simulink model "delay_test"  (R2019a)
settings: Solver=VariableStepAuto  StartTime=0.0  StopTime=512  RelTol=1e-3
libraries: xbsIndex_r4 x3559
(part 3 of 23)

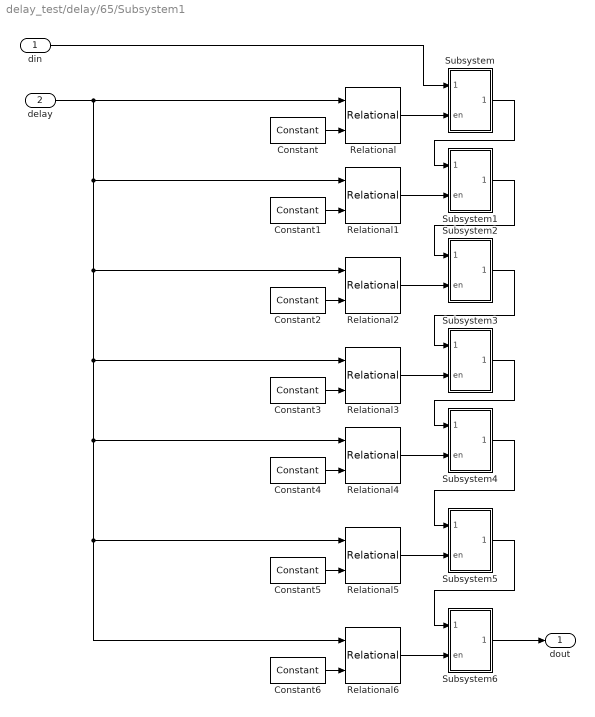
== system delay_test/delay/65/Subsystem1 ==
  din : Inport
  delay : Inport  Port=2
  Constant : xbsIndex_r4/Constant  const=0  gui_display_data_type=Fixed-point  arith_type=Unsigned  n_bits=3  bin_pt=0  preci_type=Single  exp_width=8  frac_width=24  explicit_period=on  period=1  equ=P=C  opselect=C  inp2=PCIN>>17  opr=+  inp1=P  carry=CIN  dbl_ovrd=off  block_type=constant
  Constant1 : xbsIndex_r4/Constant  const=1  gui_display_data_type=Fixed-point  arith_type=Unsigned  n_bits=3  bin_pt=0  preci_type=Single  exp_width=8  frac_width=24  explicit_period=on  period=1  equ=P=C  opselect=C  inp2=PCIN>>17  opr=+  inp1=P  carry=CIN  dbl_ovrd=off  block_type=constant
  Constant2 : xbsIndex_r4/Constant  const=2  gui_display_data_type=Fixed-point  arith_type=Unsigned  n_bits=3  bin_pt=0  preci_type=Single  exp_width=8  frac_width=24  explicit_period=on  period=1  equ=P=C  opselect=C  inp2=PCIN>>17  opr=+  inp1=P  carry=CIN  dbl_ovrd=off  block_type=constant
  Constant3 : xbsIndex_r4/Constant  const=3  gui_display_data_type=Fixed-point  arith_type=Unsigned  n_bits=3  bin_pt=0  preci_type=Single  exp_width=8  frac_width=24  explicit_period=on  period=1  equ=P=C  opselect=C  inp2=PCIN>>17  opr=+  inp1=P  carry=CIN  dbl_ovrd=off  block_type=constant
  Constant4 : xbsIndex_r4/Constant  const=4  gui_display_data_type=Fixed-point  arith_type=Unsigned  n_bits=3  bin_pt=0  preci_type=Single  exp_width=8  frac_width=24  explicit_period=on  period=1  equ=P=C  opselect=C  inp2=PCIN>>17  opr=+  inp1=P  carry=CIN  dbl_ovrd=off  block_type=constant
  Constant5 : xbsIndex_r4/Constant  const=5  gui_display_data_type=Fixed-point  arith_type=Unsigned  n_bits=3  bin_pt=0  preci_type=Single  exp_width=8  frac_width=24  explicit_period=on  period=1  equ=P=C  opselect=C  inp2=PCIN>>17  opr=+  inp1=P  carry=CIN  dbl_ovrd=off  block_type=constant
  Constant6 : xbsIndex_r4/Constant  const=6  gui_display_data_type=Fixed-point  arith_type=Unsigned  n_bits=3  bin_pt=0  preci_type=Single  exp_width=8  frac_width=24  explicit_period=on  period=1  equ=P=C  opselect=C  inp2=PCIN>>17  opr=+  inp1=P  carry=CIN  dbl_ovrd=off  block_type=constant
  Relational{,1..6} (7 alike) : xbsIndex_r4/Relational  mode=a>b  op_type=Bool  en=off  latency=1  dbl_ovrd=off  block_type=relational
  Subsystem : Subsystem
  Subsystem1 : Subsystem
  Subsystem2 : Subsystem
  Subsystem3 : Subsystem
  Subsystem4 : Subsystem
  Subsystem5 : Subsystem
  Subsystem6 : Subsystem
  dout : Outport
  wires:
  Constant3/1 -> Relational3/2
  Constant6/1 -> Relational6/2
  Constant1/1 -> Relational1/2
  Relational/1 -> Subsystem/2(en)
  Constant5/1 -> Relational5/2
  Relational1/1 -> Subsystem1/2(en)
  delay/1 -> Relational6/1, Relational5/1, Relational4/1, Relational3/1, Relational2/1, Relational1/1, Relational/1
  Constant4/1 -> Relational4/2
  Relational4/1 -> Subsystem4/2(en)
  Relational2/1 -> Subsystem2/2(en)
  Relational6/1 -> Subsystem6/2(en)
  Constant/1 -> Relational/2
  Relational5/1 -> Subsystem5/2(en)
  Relational3/1 -> Subsystem3/2(en)
  Constant2/1 -> Relational2/2
  Subsystem6/1(dout) -> dout/1
  Subsystem4/1(dout) -> Subsystem5/1(din)
  Subsystem5/1(dout) -> Subsystem6/1(din)
  Subsystem3/1(dout) -> Subsystem4/1(din)
  Subsystem2/1(dout) -> Subsystem3/1(din)
  Subsystem1/1(dout) -> Subsystem2/1(din)
  Subsystem/1(dout) -> Subsystem1/1(din)
  din/1 -> Subsystem/1(din)

== system delay_test/delay/65/delay ==
  sim_1 : Inport
  io_delay : xbsIndex_r4/Delay  rst=off  infoeditControl=Selection of Reset will increase slice count due to use of real FFs and instead of SRLs  en=off  latency=0  reg_retiming=on  dbl_ovrd=off  block_type=delay
  reint1 : xbsIndex_r4/Reinterpret  force_arith_type=on  arith_type=Unsigned  force_bin_pt=on  bin_pt=0  block_type=reinterpret
  slice_reg : xbsIndex_r4/Slice  nbits=13  boolean_output=off  mode=Lower Bit Location + Width  bit1=0  base1=MSB of Input  bit0=0  base0=LSB of Input  dbl_ovrd=off  block_type=slice
  snap2_f_200msps_64i_4096c_delay_0_delay_user_data_out : xbsIndex_r4/Gateway In  gui_display_data_type=Fixed-point  arith_type=Unsigned  n_bits=32  bin_pt=0  preci_type=Single  exp_width=8  frac_width=24  rows=1  columns=1  quantization="Round  (unbiased: +/- Inf)"  overflow=Saturate  period=1  UseAsADC=off  ADCChannel='1'  interface=None  automatic_assignment=on  address_offset=hex2dec('00')  intf_name=''  intf_description=''  default_value=0  timing_constraint=None  locs_specified=off  LOCs={}  io_standard={}  inherit_from_input=off  hdl_port=on  dbl_ovrd=off  block_type=gatewayin
  in_reg : Outport
  wires:
  reint1/1 -> in_reg/1
  slice_reg/1 -> reint1/1
  io_delay/1 -> slice_reg/1
  ? -> snap2_f_200msps_64i_4096c_delay_0_delay_user_data_out/1
  ? -> ?
  ? -> ?
  sim_1/1 -> ?
  snap2_f_200msps_64i_4096c_delay_0_delay_user_data_out/1 -> io_delay/1

== system delay_test/delay/65/delay_bram_prog_dp ==
  din : Inport
  delay : Inport  Port=2
  AddSub : xbsIndex_r4/AddSub  mode=Subtraction  use_carryin=off  use_carryout=off  en=off  latency=1  precision=User Defined  arith_type=Unsigned  n_bits=ram_bits  bin_pt=0  quantization=Truncate  overflow=Wrap  use_behavioral_HDL=on  hw_selection=Fabric  pipelined=off  use_rpm=on  dbl_ovrd=off  block_type=addsub
  Constant2 : xbsIndex_r4/Constant  const=1.0  gui_display_data_type=Fixed-point  arith_type=Boolean  n_bits=1  bin_pt=0  preci_type=Single  exp_width=8  frac_width=24  explicit_period=on  period=1  equ=P=C  opselect=C  inp2=PCIN>>17  opr=+  inp1=P  carry=CIN  dbl_ovrd=off  block_type=constant
  Constant4 : xbsIndex_r4/Constant  const=0  gui_display_data_type=Fixed-point  arith_type=Boolean  n_bits=1  bin_pt=0  preci_type=Single  exp_width=8  frac_width=24  explicit_period=on  period=1  equ=P=C  opselect=C  inp2=PCIN>>17  opr=+  inp1=P  carry=CIN  dbl_ovrd=off  block_type=constant
  Dual Port RAM : xbsIndex_r4/Dual Port RAM  depth=2^ram_bits  initVector=0  distributed_mem=Block RAM  init_a=0  init_b=0  rst_a=off  rst_b=off  en_a=off  en_b=off  latency=bram_latency  write_mode_A=Read After Write  write_mode_B=Read Before Write  optimize=Area  dbl_ovrd=off  block_type=dpram
  Terminator : Terminator
  wr_addr : xbsIndex_r4/Counter  cnt_type=Free Running  cnt_to=Inf  operation=Up  start_count=0  cnt_by_val=1  arith_type=Unsigned  n_bits=ram_bits  bin_pt=0  load_pin=off  rst=off  en=off  explicit_period=on  period=1  use_behavioral_HDL=on  implementation=Fabric  use_rpm=on  dbl_ovrd=off  block_type=counter
  dout : Outport
  wires:
  Dual Port RAM/2 -> dout/1
  Dual Port RAM/1 -> Terminator/1
  Constant4/1 -> Dual Port RAM/6
  Constant2/1 -> Dual Port RAM/3
  AddSub/1 -> Dual Port RAM/4
  din/1 -> Dual Port RAM/5, Dual Port RAM/2
  wr_addr/1 -> Dual Port RAM/1, AddSub/1
  delay/1 -> AddSub/2

== system delay_test/delay/Subsystem/0 ==
  din : Inport
  delay : Inport  Port=2
  Slice : xbsIndex_r4/Slice  nbits=10  boolean_output=off  mode=Lower Bit Location + Width  bit1=0  base1=MSB of Input  bit0=0  base0=LSB of Input  dbl_ovrd=off  block_type=slice
  Slice1 : xbsIndex_r4/Slice  nbits=3  boolean_output=off  mode=Lower Bit Location + Width  bit1=0  base1=MSB of Input  bit0=10  base0=LSB of Input  dbl_ovrd=off  block_type=slice
  Subsystem1 : Subsystem
  delay_bram_prog_dp : Subsystem  AncestorBlock=casper_library_delays/delay_bram_prog_dp  mask(delay_bram_prog_dp){ram_bits=max_delay_bits-3, bram_latency=2, async=off}
      mask prompts: ram_bits "Max delay (2^?)"; bram_latency "BRAM latency"; async "asynchronous operation"
      mask init:
      | delay_bram_prog_dp_init(gcb, ...
      |     'ram_bits', ram_bits, ...
      |     'bram_latency', bram_latency, ...
      |     'async', async);
  dout : Outport
  wires:
  Subsystem1/1(dout) -> dout/1
  delay_bram_prog_dp/1(dout) -> Subsystem1/1(din)
  Slice1/1 -> Subsystem1/2(delay)
  Slice/1 -> delay_bram_prog_dp/2(delay)
  delay/1 -> Slice/1, Slice1/1
  din/1 -> delay_bram_prog_dp/1(din)

== system delay_test/delay/Subsystem/1 ==
  din : Inport
  delay : Inport  Port=2
  Slice : xbsIndex_r4/Slice  nbits=10  boolean_output=off  mode=Lower Bit Location + Width  bit1=0  base1=MSB of Input  bit0=0  base0=LSB of Input  dbl_ovrd=off  block_type=slice
  Slice1 : xbsIndex_r4/Slice  nbits=3  boolean_output=off  mode=Lower Bit Location + Width  bit1=0  base1=MSB of Input  bit0=10  base0=LSB of Input  dbl_ovrd=off  block_type=slice
  Subsystem1 : Subsystem
  delay_bram_prog_dp : Subsystem  AncestorBlock=casper_library_delays/delay_bram_prog_dp  mask(delay_bram_prog_dp){ram_bits=max_delay_bits-3, bram_latency=2, async=off}
      mask prompts: ram_bits "Max delay (2^?)"; bram_latency "BRAM latency"; async "asynchronous operation"
      mask init:
      | delay_bram_prog_dp_init(gcb, ...
      |     'ram_bits', ram_bits, ...
      |     'bram_latency', bram_latency, ...
      |     'async', async);
  dout : Outport
  wires:
  din/1 -> delay_bram_prog_dp/1(din)
  delay/1 -> Slice1/1, Slice/1
  Slice/1 -> delay_bram_prog_dp/2(delay)
  Slice1/1 -> Subsystem1/2(delay)
  delay_bram_prog_dp/1(dout) -> Subsystem1/1(din)
  Subsystem1/1(dout) -> dout/1

== system delay_test/delay/Subsystem/10 ==
  din : Inport
  delay : Inport  Port=2
  Slice : xbsIndex_r4/Slice  nbits=10  boolean_output=off  mode=Lower Bit Location + Width  bit1=0  base1=MSB of Input  bit0=0  base0=LSB of Input  dbl_ovrd=off  block_type=slice
  Slice1 : xbsIndex_r4/Slice  nbits=3  boolean_output=off  mode=Lower Bit Location + Width  bit1=0  base1=MSB of Input  bit0=10  base0=LSB of Input  dbl_ovrd=off  block_type=slice
  Subsystem1 : Subsystem
  delay_bram_prog_dp : Subsystem  AncestorBlock=casper_library_delays/delay_bram_prog_dp  mask(delay_bram_prog_dp){ram_bits=max_delay_bits-3, bram_latency=2, async=off}
      mask prompts: ram_bits "Max delay (2^?)"; bram_latency "BRAM latency"; async "asynchronous operation"
      mask init:
      | delay_bram_prog_dp_init(gcb, ...
      |     'ram_bits', ram_bits, ...
      |     'bram_latency', bram_latency, ...
      |     'async', async);
  dout : Outport
  wires:
  Subsystem1/1(dout) -> dout/1
  delay_bram_prog_dp/1(dout) -> Subsystem1/1(din)
  Slice1/1 -> Subsystem1/2(delay)
  Slice/1 -> delay_bram_prog_dp/2(delay)
  delay/1 -> Slice/1, Slice1/1
  din/1 -> delay_bram_prog_dp/1(din)

== system delay_test/delay/Subsystem/11 ==
  din : Inport
  delay : Inport  Port=2
  Slice : xbsIndex_r4/Slice  nbits=10  boolean_output=off  mode=Lower Bit Location + Width  bit1=0  base1=MSB of Input  bit0=0  base0=LSB of Input  dbl_ovrd=off  block_type=slice
  Slice1 : xbsIndex_r4/Slice  nbits=3  boolean_output=off  mode=Lower Bit Location + Width  bit1=0  base1=MSB of Input  bit0=10  base0=LSB of Input  dbl_ovrd=off  block_type=slice
  Subsystem1 : Subsystem
  delay_bram_prog_dp : Subsystem  AncestorBlock=casper_library_delays/delay_bram_prog_dp  mask(delay_bram_prog_dp){ram_bits=max_delay_bits-3, bram_latency=2, async=off}
      mask prompts: ram_bits "Max delay (2^?)"; bram_latency "BRAM latency"; async "asynchronous operation"
      mask init:
      | delay_bram_prog_dp_init(gcb, ...
      |     'ram_bits', ram_bits, ...
      |     'bram_latency', bram_latency, ...
      |     'async', async);
  dout : Outport
  wires:
  din/1 -> delay_bram_prog_dp/1(din)
  delay/1 -> Slice1/1, Slice/1
  Slice/1 -> delay_bram_prog_dp/2(delay)
  Slice1/1 -> Subsystem1/2(delay)
  delay_bram_prog_dp/1(dout) -> Subsystem1/1(din)
  Subsystem1/1(dout) -> dout/1

== system delay_test/delay/Subsystem/12 ==
  din : Inport
  delay : Inport  Port=2
  Slice : xbsIndex_r4/Slice  nbits=10  boolean_output=off  mode=Lower Bit Location + Width  bit1=0  base1=MSB of Input  bit0=0  base0=LSB of Input  dbl_ovrd=off  block_type=slice
  Slice1 : xbsIndex_r4/Slice  nbits=3  boolean_output=off  mode=Lower Bit Location + Width  bit1=0  base1=MSB of Input  bit0=10  base0=LSB of Input  dbl_ovrd=off  block_type=slice
  Subsystem1 : Subsystem
  delay_bram_prog_dp : Subsystem  AncestorBlock=casper_library_delays/delay_bram_prog_dp  mask(delay_bram_prog_dp){ram_bits=max_delay_bits-3, bram_latency=2, async=off}
      mask prompts: ram_bits "Max delay (2^?)"; bram_latency "BRAM latency"; async "asynchronous operation"
      mask init:
      | delay_bram_prog_dp_init(gcb, ...
      |     'ram_bits', ram_bits, ...
      |     'bram_latency', bram_latency, ...
      |     'async', async);
  dout : Outport
  wires:
  Subsystem1/1(dout) -> dout/1
  delay_bram_prog_dp/1(dout) -> Subsystem1/1(din)
  Slice1/1 -> Subsystem1/2(delay)
  Slice/1 -> delay_bram_prog_dp/2(delay)
  delay/1 -> Slice/1, Slice1/1
  din/1 -> delay_bram_prog_dp/1(din)

== system delay_test/delay/Subsystem/13 ==
  din : Inport
  delay : Inport  Port=2
  Slice : xbsIndex_r4/Slice  nbits=10  boolean_output=off  mode=Lower Bit Location + Width  bit1=0  base1=MSB of Input  bit0=0  base0=LSB of Input  dbl_ovrd=off  block_type=slice
  Slice1 : xbsIndex_r4/Slice  nbits=3  boolean_output=off  mode=Lower Bit Location + Width  bit1=0  base1=MSB of Input  bit0=10  base0=LSB of Input  dbl_ovrd=off  block_type=slice
  Subsystem1 : Subsystem
  delay_bram_prog_dp : Subsystem  AncestorBlock=casper_library_delays/delay_bram_prog_dp  mask(delay_bram_prog_dp){ram_bits=max_delay_bits-3, bram_latency=2, async=off}
      mask prompts: ram_bits "Max delay (2^?)"; bram_latency "BRAM latency"; async "asynchronous operation"
      mask init:
      | delay_bram_prog_dp_init(gcb, ...
      |     'ram_bits', ram_bits, ...
      |     'bram_latency', bram_latency, ...
      |     'async', async);
  dout : Outport
  wires:
  din/1 -> delay_bram_prog_dp/1(din)
  delay/1 -> Slice1/1, Slice/1
  Slice/1 -> delay_bram_prog_dp/2(delay)
  Slice1/1 -> Subsystem1/2(delay)
  delay_bram_prog_dp/1(dout) -> Subsystem1/1(din)
  Subsystem1/1(dout) -> dout/1

== system delay_test/delay/Subsystem/14 ==
  din : Inport
  delay : Inport  Port=2
  Slice : xbsIndex_r4/Slice  nbits=10  boolean_output=off  mode=Lower Bit Location + Width  bit1=0  base1=MSB of Input  bit0=0  base0=LSB of Input  dbl_ovrd=off  block_type=slice
  Slice1 : xbsIndex_r4/Slice  nbits=3  boolean_output=off  mode=Lower Bit Location + Width  bit1=0  base1=MSB of Input  bit0=10  base0=LSB of Input  dbl_ovrd=off  block_type=slice
  Subsystem1 : Subsystem
  delay_bram_prog_dp : Subsystem  AncestorBlock=casper_library_delays/delay_bram_prog_dp  mask(delay_bram_prog_dp){ram_bits=max_delay_bits-3, bram_latency=2, async=off}
      mask prompts: ram_bits "Max delay (2^?)"; bram_latency "BRAM latency"; async "asynchronous operation"
      mask init:
      | delay_bram_prog_dp_init(gcb, ...
      |     'ram_bits', ram_bits, ...
      |     'bram_latency', bram_latency, ...
      |     'async', async);
  dout : Outport
  wires:
  din/1 -> delay_bram_prog_dp/1(din)
  delay/1 -> Slice1/1, Slice/1
  Slice/1 -> delay_bram_prog_dp/2(delay)
  Slice1/1 -> Subsystem1/2(delay)
  delay_bram_prog_dp/1(dout) -> Subsystem1/1(din)
  Subsystem1/1(dout) -> dout/1

== system delay_test/delay/Subsystem/15 ==
  din : Inport
  delay : Inport  Port=2
  Slice : xbsIndex_r4/Slice  nbits=10  boolean_output=off  mode=Lower Bit Location + Width  bit1=0  base1=MSB of Input  bit0=0  base0=LSB of Input  dbl_ovrd=off  block_type=slice
  Slice1 : xbsIndex_r4/Slice  nbits=3  boolean_output=off  mode=Lower Bit Location + Width  bit1=0  base1=MSB of Input  bit0=10  base0=LSB of Input  dbl_ovrd=off  block_type=slice
  Subsystem1 : Subsystem
  delay_bram_prog_dp : Subsystem  AncestorBlock=casper_library_delays/delay_bram_prog_dp  mask(delay_bram_prog_dp){ram_bits=max_delay_bits-3, bram_latency=2, async=off}
      mask prompts: ram_bits "Max delay (2^?)"; bram_latency "BRAM latency"; async "asynchronous operation"
      mask init:
      | delay_bram_prog_dp_init(gcb, ...
      |     'ram_bits', ram_bits, ...
      |     'bram_latency', bram_latency, ...
      |     'async', async);
  dout : Outport
  wires:
  Subsystem1/1(dout) -> dout/1
  delay_bram_prog_dp/1(dout) -> Subsystem1/1(din)
  Slice1/1 -> Subsystem1/2(delay)
  Slice/1 -> delay_bram_prog_dp/2(delay)
  delay/1 -> Slice/1, Slice1/1
  din/1 -> delay_bram_prog_dp/1(din)

== system delay_test/delay/Subsystem/16 ==
  din : Inport
  delay : Inport  Port=2
  Slice : xbsIndex_r4/Slice  nbits=10  boolean_output=off  mode=Lower Bit Location + Width  bit1=0  base1=MSB of Input  bit0=0  base0=LSB of Input  dbl_ovrd=off  block_type=slice
  Slice1 : xbsIndex_r4/Slice  nbits=3  boolean_output=off  mode=Lower Bit Location + Width  bit1=0  base1=MSB of Input  bit0=10  base0=LSB of Input  dbl_ovrd=off  block_type=slice
  Subsystem1 : Subsystem
  delay_bram_prog_dp : Subsystem  AncestorBlock=casper_library_delays/delay_bram_prog_dp  mask(delay_bram_prog_dp){ram_bits=max_delay_bits-3, bram_latency=2, async=off}
      mask prompts: ram_bits "Max delay (2^?)"; bram_latency "BRAM latency"; async "asynchronous operation"
      mask init:
      | delay_bram_prog_dp_init(gcb, ...
      |     'ram_bits', ram_bits, ...
      |     'bram_latency', bram_latency, ...
      |     'async', async);
  dout : Outport
  wires:
  din/1 -> delay_bram_prog_dp/1(din)
  delay/1 -> Slice1/1, Slice/1
  Slice/1 -> delay_bram_prog_dp/2(delay)
  Slice1/1 -> Subsystem1/2(delay)
  delay_bram_prog_dp/1(dout) -> Subsystem1/1(din)
  Subsystem1/1(dout) -> dout/1

== system delay_test/delay/Subsystem/17 ==
  din : Inport
  delay : Inport  Port=2
  Slice : xbsIndex_r4/Slice  nbits=10  boolean_output=off  mode=Lower Bit Location + Width  bit1=0  base1=MSB of Input  bit0=0  base0=LSB of Input  dbl_ovrd=off  block_type=slice
  Slice1 : xbsIndex_r4/Slice  nbits=3  boolean_output=off  mode=Lower Bit Location + Width  bit1=0  base1=MSB of Input  bit0=10  base0=LSB of Input  dbl_ovrd=off  block_type=slice
  Subsystem1 : Subsystem
  delay_bram_prog_dp : Subsystem  AncestorBlock=casper_library_delays/delay_bram_prog_dp  mask(delay_bram_prog_dp){ram_bits=max_delay_bits-3, bram_latency=2, async=off}
      mask prompts: ram_bits "Max delay (2^?)"; bram_latency "BRAM latency"; async "asynchronous operation"
      mask init:
      | delay_bram_prog_dp_init(gcb, ...
      |     'ram_bits', ram_bits, ...
      |     'bram_latency', bram_latency, ...
      |     'async', async);
  dout : Outport
  wires:
  Subsystem1/1(dout) -> dout/1
  delay_bram_prog_dp/1(dout) -> Subsystem1/1(din)
  Slice1/1 -> Subsystem1/2(delay)
  Slice/1 -> delay_bram_prog_dp/2(delay)
  delay/1 -> Slice/1, Slice1/1
  din/1 -> delay_bram_prog_dp/1(din)

== system delay_test/delay/Subsystem/18 ==
  din : Inport
  delay : Inport  Port=2
  Slice : xbsIndex_r4/Slice  nbits=10  boolean_output=off  mode=Lower Bit Location + Width  bit1=0  base1=MSB of Input  bit0=0  base0=LSB of Input  dbl_ovrd=off  block_type=slice
  Slice1 : xbsIndex_r4/Slice  nbits=3  boolean_output=off  mode=Lower Bit Location + Width  bit1=0  base1=MSB of Input  bit0=10  base0=LSB of Input  dbl_ovrd=off  block_type=slice
  Subsystem1 : Subsystem
  delay_bram_prog_dp : Subsystem  AncestorBlock=casper_library_delays/delay_bram_prog_dp  mask(delay_bram_prog_dp){ram_bits=max_delay_bits-3, bram_latency=2, async=off}
      mask prompts: ram_bits "Max delay (2^?)"; bram_latency "BRAM latency"; async "asynchronous operation"
      mask init:
      | delay_bram_prog_dp_init(gcb, ...
      |     'ram_bits', ram_bits, ...
      |     'bram_latency', bram_latency, ...
      |     'async', async);
  dout : Outport
  wires:
  din/1 -> delay_bram_prog_dp/1(din)
  delay/1 -> Slice1/1, Slice/1
  Slice/1 -> delay_bram_prog_dp/2(delay)
  Slice1/1 -> Subsystem1/2(delay)
  delay_bram_prog_dp/1(dout) -> Subsystem1/1(din)
  Subsystem1/1(dout) -> dout/1

== system delay_test/delay/Subsystem/19 ==
  din : Inport
  delay : Inport  Port=2
  Slice : xbsIndex_r4/Slice  nbits=10  boolean_output=off  mode=Lower Bit Location + Width  bit1=0  base1=MSB of Input  bit0=0  base0=LSB of Input  dbl_ovrd=off  block_type=slice
  Slice1 : xbsIndex_r4/Slice  nbits=3  boolean_output=off  mode=Lower Bit Location + Width  bit1=0  base1=MSB of Input  bit0=10  base0=LSB of Input  dbl_ovrd=off  block_type=slice
  Subsystem1 : Subsystem
  delay_bram_prog_dp : Subsystem  AncestorBlock=casper_library_delays/delay_bram_prog_dp  mask(delay_bram_prog_dp){ram_bits=max_delay_bits-3, bram_latency=2, async=off}
      mask prompts: ram_bits "Max delay (2^?)"; bram_latency "BRAM latency"; async "asynchronous operation"
      mask init:
      | delay_bram_prog_dp_init(gcb, ...
      |     'ram_bits', ram_bits, ...
      |     'bram_latency', bram_latency, ...
      |     'async', async);
  dout : Outport
  wires:
  Subsystem1/1(dout) -> dout/1
  delay_bram_prog_dp/1(dout) -> Subsystem1/1(din)
  Slice1/1 -> Subsystem1/2(delay)
  Slice/1 -> delay_bram_prog_dp/2(delay)
  delay/1 -> Slice/1, Slice1/1
  din/1 -> delay_bram_prog_dp/1(din)

== system delay_test/delay/Subsystem/2 ==
  din : Inport
  delay : Inport  Port=2
  Slice : xbsIndex_r4/Slice  nbits=10  boolean_output=off  mode=Lower Bit Location + Width  bit1=0  base1=MSB of Input  bit0=0  base0=LSB of Input  dbl_ovrd=off  block_type=slice
  Slice1 : xbsIndex_r4/Slice  nbits=3  boolean_output=off  mode=Lower Bit Location + Width  bit1=0  base1=MSB of Input  bit0=10  base0=LSB of Input  dbl_ovrd=off  block_type=slice
  Subsystem1 : Subsystem
  delay_bram_prog_dp : Subsystem  AncestorBlock=casper_library_delays/delay_bram_prog_dp  mask(delay_bram_prog_dp){ram_bits=max_delay_bits-3, bram_latency=2, async=off}
      mask prompts: ram_bits "Max delay (2^?)"; bram_latency "BRAM latency"; async "asynchronous operation"
      mask init:
      | delay_bram_prog_dp_init(gcb, ...
      |     'ram_bits', ram_bits, ...
      |     'bram_latency', bram_latency, ...
      |     'async', async);
  dout : Outport
  wires:
  din/1 -> delay_bram_prog_dp/1(din)
  delay/1 -> Slice1/1, Slice/1
  Slice/1 -> delay_bram_prog_dp/2(delay)
  Slice1/1 -> Subsystem1/2(delay)
  delay_bram_prog_dp/1(dout) -> Subsystem1/1(din)
  Subsystem1/1(dout) -> dout/1

== system delay_test/delay/Subsystem/20 ==
  din : Inport
  delay : Inport  Port=2
  Slice : xbsIndex_r4/Slice  nbits=10  boolean_output=off  mode=Lower Bit Location + Width  bit1=0  base1=MSB of Input  bit0=0  base0=LSB of Input  dbl_ovrd=off  block_type=slice
  Slice1 : xbsIndex_r4/Slice  nbits=3  boolean_output=off  mode=Lower Bit Location + Width  bit1=0  base1=MSB of Input  bit0=10  base0=LSB of Input  dbl_ovrd=off  block_type=slice
  Subsystem1 : Subsystem
  delay_bram_prog_dp : Subsystem  AncestorBlock=casper_library_delays/delay_bram_prog_dp  mask(delay_bram_prog_dp){ram_bits=max_delay_bits-3, bram_latency=2, async=off}
      mask prompts: ram_bits "Max delay (2^?)"; bram_latency "BRAM latency"; async "asynchronous operation"
      mask init:
      | delay_bram_prog_dp_init(gcb, ...
      |     'ram_bits', ram_bits, ...
      |     'bram_latency', bram_latency, ...
      |     'async', async);
  dout : Outport
  wires:
  Subsystem1/1(dout) -> dout/1
  delay_bram_prog_dp/1(dout) -> Subsystem1/1(din)
  Slice1/1 -> Subsystem1/2(delay)
  Slice/1 -> delay_bram_prog_dp/2(delay)
  delay/1 -> Slice/1, Slice1/1
  din/1 -> delay_bram_prog_dp/1(din)

== system delay_test/delay/Subsystem/21 ==
  din : Inport
  delay : Inport  Port=2
  Slice : xbsIndex_r4/Slice  nbits=10  boolean_output=off  mode=Lower Bit Location + Width  bit1=0  base1=MSB of Input  bit0=0  base0=LSB of Input  dbl_ovrd=off  block_type=slice
  Slice1 : xbsIndex_r4/Slice  nbits=3  boolean_output=off  mode=Lower Bit Location + Width  bit1=0  base1=MSB of Input  bit0=10  base0=LSB of Input  dbl_ovrd=off  block_type=slice
  Subsystem1 : Subsystem
  delay_bram_prog_dp : Subsystem  AncestorBlock=casper_library_delays/delay_bram_prog_dp  mask(delay_bram_prog_dp){ram_bits=max_delay_bits-3, bram_latency=2, async=off}
      mask prompts: ram_bits "Max delay (2^?)"; bram_latency "BRAM latency"; async "asynchronous operation"
      mask init:
      | delay_bram_prog_dp_init(gcb, ...
      |     'ram_bits', ram_bits, ...
      |     'bram_latency', bram_latency, ...
      |     'async', async);
  dout : Outport
  wires:
  din/1 -> delay_bram_prog_dp/1(din)
  delay/1 -> Slice1/1, Slice/1
  Slice/1 -> delay_bram_prog_dp/2(delay)
  Slice1/1 -> Subsystem1/2(delay)
  delay_bram_prog_dp/1(dout) -> Subsystem1/1(din)
  Subsystem1/1(dout) -> dout/1

== system delay_test/delay/Subsystem/22 ==
  din : Inport
  delay : Inport  Port=2
  Slice : xbsIndex_r4/Slice  nbits=10  boolean_output=off  mode=Lower Bit Location + Width  bit1=0  base1=MSB of Input  bit0=0  base0=LSB of Input  dbl_ovrd=off  block_type=slice
  Slice1 : xbsIndex_r4/Slice  nbits=3  boolean_output=off  mode=Lower Bit Location + Width  bit1=0  base1=MSB of Input  bit0=10  base0=LSB of Input  dbl_ovrd=off  block_type=slice
  Subsystem1 : Subsystem
  delay_bram_prog_dp : Subsystem  AncestorBlock=casper_library_delays/delay_bram_prog_dp  mask(delay_bram_prog_dp){ram_bits=max_delay_bits-3, bram_latency=2, async=off}
      mask prompts: ram_bits "Max delay (2^?)"; bram_latency "BRAM latency"; async "asynchronous operation"
      mask init:
      | delay_bram_prog_dp_init(gcb, ...
      |     'ram_bits', ram_bits, ...
      |     'bram_latency', bram_latency, ...
      |     'async', async);
  dout : Outport
  wires:
  Subsystem1/1(dout) -> dout/1
  delay_bram_prog_dp/1(dout) -> Subsystem1/1(din)
  Slice1/1 -> Subsystem1/2(delay)
  Slice/1 -> delay_bram_prog_dp/2(delay)
  delay/1 -> Slice/1, Slice1/1
  din/1 -> delay_bram_prog_dp/1(din)

== system delay_test/delay/Subsystem/23 ==
  din : Inport
  delay : Inport  Port=2
  Slice : xbsIndex_r4/Slice  nbits=10  boolean_output=off  mode=Lower Bit Location + Width  bit1=0  base1=MSB of Input  bit0=0  base0=LSB of Input  dbl_ovrd=off  block_type=slice
  Slice1 : xbsIndex_r4/Slice  nbits=3  boolean_output=off  mode=Lower Bit Location + Width  bit1=0  base1=MSB of Input  bit0=10  base0=LSB of Input  dbl_ovrd=off  block_type=slice
  Subsystem1 : Subsystem
  delay_bram_prog_dp : Subsystem  AncestorBlock=casper_library_delays/delay_bram_prog_dp  mask(delay_bram_prog_dp){ram_bits=max_delay_bits-3, bram_latency=2, async=off}
      mask prompts: ram_bits "Max delay (2^?)"; bram_latency "BRAM latency"; async "asynchronous operation"
      mask init:
      | delay_bram_prog_dp_init(gcb, ...
      |     'ram_bits', ram_bits, ...
      |     'bram_latency', bram_latency, ...
      |     'async', async);
  dout : Outport
  wires:
  din/1 -> delay_bram_prog_dp/1(din)
  delay/1 -> Slice1/1, Slice/1
  Slice/1 -> delay_bram_prog_dp/2(delay)
  Slice1/1 -> Subsystem1/2(delay)
  delay_bram_prog_dp/1(dout) -> Subsystem1/1(din)
  Subsystem1/1(dout) -> dout/1

== system delay_test/delay/Subsystem/24 ==
  din : Inport
  delay : Inport  Port=2
  Slice : xbsIndex_r4/Slice  nbits=10  boolean_output=off  mode=Lower Bit Location + Width  bit1=0  base1=MSB of Input  bit0=0  base0=LSB of Input  dbl_ovrd=off  block_type=slice
  Slice1 : xbsIndex_r4/Slice  nbits=3  boolean_output=off  mode=Lower Bit Location + Width  bit1=0  base1=MSB of Input  bit0=10  base0=LSB of Input  dbl_ovrd=off  block_type=slice
  Subsystem1 : Subsystem
  delay_bram_prog_dp : Subsystem  AncestorBlock=casper_library_delays/delay_bram_prog_dp  mask(delay_bram_prog_dp){ram_bits=max_delay_bits-3, bram_latency=2, async=off}
      mask prompts: ram_bits "Max delay (2^?)"; bram_latency "BRAM latency"; async "asynchronous operation"
      mask init:
      | delay_bram_prog_dp_init(gcb, ...
      |     'ram_bits', ram_bits, ...
      |     'bram_latency', bram_latency, ...
      |     'async', async);
  dout : Outport
  wires:
  Subsystem1/1(dout) -> dout/1
  delay_bram_prog_dp/1(dout) -> Subsystem1/1(din)
  Slice1/1 -> Subsystem1/2(delay)
  Slice/1 -> delay_bram_prog_dp/2(delay)
  delay/1 -> Slice/1, Slice1/1
  din/1 -> delay_bram_prog_dp/1(din)

== system delay_test/delay/Subsystem/25 ==
  din : Inport
  delay : Inport  Port=2
  Slice : xbsIndex_r4/Slice  nbits=10  boolean_output=off  mode=Lower Bit Location + Width  bit1=0  base1=MSB of Input  bit0=0  base0=LSB of Input  dbl_ovrd=off  block_type=slice
  Slice1 : xbsIndex_r4/Slice  nbits=3  boolean_output=off  mode=Lower Bit Location + Width  bit1=0  base1=MSB of Input  bit0=10  base0=LSB of Input  dbl_ovrd=off  block_type=slice
  Subsystem1 : Subsystem
  delay_bram_prog_dp : Subsystem  AncestorBlock=casper_library_delays/delay_bram_prog_dp  mask(delay_bram_prog_dp){ram_bits=max_delay_bits-3, bram_latency=2, async=off}
      mask prompts: ram_bits "Max delay (2^?)"; bram_latency "BRAM latency"; async "asynchronous operation"
      mask init:
      | delay_bram_prog_dp_init(gcb, ...
      |     'ram_bits', ram_bits, ...
      |     'bram_latency', bram_latency, ...
      |     'async', async);
  dout : Outport
  wires:
  din/1 -> delay_bram_prog_dp/1(din)
  delay/1 -> Slice1/1, Slice/1
  Slice/1 -> delay_bram_prog_dp/2(delay)
  Slice1/1 -> Subsystem1/2(delay)
  delay_bram_prog_dp/1(dout) -> Subsystem1/1(din)
  Subsystem1/1(dout) -> dout/1

== system delay_test/delay/Subsystem/26 ==
  din : Inport
  delay : Inport  Port=2
  Slice : xbsIndex_r4/Slice  nbits=10  boolean_output=off  mode=Lower Bit Location + Width  bit1=0  base1=MSB of Input  bit0=0  base0=LSB of Input  dbl_ovrd=off  block_type=slice
  Slice1 : xbsIndex_r4/Slice  nbits=3  boolean_output=off  mode=Lower Bit Location + Width  bit1=0  base1=MSB of Input  bit0=10  base0=LSB of Input  dbl_ovrd=off  block_type=slice
  Subsystem1 : Subsystem
  delay_bram_prog_dp : Subsystem  AncestorBlock=casper_library_delays/delay_bram_prog_dp  mask(delay_bram_prog_dp){ram_bits=max_delay_bits-3, bram_latency=2, async=off}
      mask prompts: ram_bits "Max delay (2^?)"; bram_latency "BRAM latency"; async "asynchronous operation"
      mask init:
      | delay_bram_prog_dp_init(gcb, ...
      |     'ram_bits', ram_bits, ...
      |     'bram_latency', bram_latency, ...
      |     'async', async);
  dout : Outport
  wires:
  Subsystem1/1(dout) -> dout/1
  delay_bram_prog_dp/1(dout) -> Subsystem1/1(din)
  Slice1/1 -> Subsystem1/2(delay)
  Slice/1 -> delay_bram_prog_dp/2(delay)
  delay/1 -> Slice/1, Slice1/1
  din/1 -> delay_bram_prog_dp/1(din)

== system delay_test/delay/Subsystem/27 ==
  din : Inport
  delay : Inport  Port=2
  Slice : xbsIndex_r4/Slice  nbits=10  boolean_output=off  mode=Lower Bit Location + Width  bit1=0  base1=MSB of Input  bit0=0  base0=LSB of Input  dbl_ovrd=off  block_type=slice
  Slice1 : xbsIndex_r4/Slice  nbits=3  boolean_output=off  mode=Lower Bit Location + Width  bit1=0  base1=MSB of Input  bit0=10  base0=LSB of Input  dbl_ovrd=off  block_type=slice
  Subsystem1 : Subsystem
  delay_bram_prog_dp : Subsystem  AncestorBlock=casper_library_delays/delay_bram_prog_dp  mask(delay_bram_prog_dp){ram_bits=max_delay_bits-3, bram_latency=2, async=off}
      mask prompts: ram_bits "Max delay (2^?)"; bram_latency "BRAM latency"; async "asynchronous operation"
      mask init:
      | delay_bram_prog_dp_init(gcb, ...
      |     'ram_bits', ram_bits, ...
      |     'bram_latency', bram_latency, ...
      |     'async', async);
  dout : Outport
  wires:
  din/1 -> delay_bram_prog_dp/1(din)
  delay/1 -> Slice1/1, Slice/1
  Slice/1 -> delay_bram_prog_dp/2(delay)
  Slice1/1 -> Subsystem1/2(delay)
  delay_bram_prog_dp/1(dout) -> Subsystem1/1(din)
  Subsystem1/1(dout) -> dout/1

== system delay_test/delay/Subsystem/28 ==
  din : Inport
  delay : Inport  Port=2
  Slice : xbsIndex_r4/Slice  nbits=10  boolean_output=off  mode=Lower Bit Location + Width  bit1=0  base1=MSB of Input  bit0=0  base0=LSB of Input  dbl_ovrd=off  block_type=slice
  Slice1 : xbsIndex_r4/Slice  nbits=3  boolean_output=off  mode=Lower Bit Location + Width  bit1=0  base1=MSB of Input  bit0=10  base0=LSB of Input  dbl_ovrd=off  block_type=slice
  Subsystem1 : Subsystem
  delay_bram_prog_dp : Subsystem  AncestorBlock=casper_library_delays/delay_bram_prog_dp  mask(delay_bram_prog_dp){ram_bits=max_delay_bits-3, bram_latency=2, async=off}
      mask prompts: ram_bits "Max delay (2^?)"; bram_latency "BRAM latency"; async "asynchronous operation"
      mask init:
      | delay_bram_prog_dp_init(gcb, ...
      |     'ram_bits', ram_bits, ...
      |     'bram_latency', bram_latency, ...
      |     'async', async);
  dout : Outport
  wires:
  din/1 -> delay_bram_prog_dp/1(din)
  delay/1 -> Slice1/1, Slice/1
  Slice/1 -> delay_bram_prog_dp/2(delay)
  Slice1/1 -> Subsystem1/2(delay)
  delay_bram_prog_dp/1(dout) -> Subsystem1/1(din)
  Subsystem1/1(dout) -> dout/1

== system delay_test/delay/Subsystem/29 ==
  din : Inport
  delay : Inport  Port=2
  Slice : xbsIndex_r4/Slice  nbits=10  boolean_output=off  mode=Lower Bit Location + Width  bit1=0  base1=MSB of Input  bit0=0  base0=LSB of Input  dbl_ovrd=off  block_type=slice
  Slice1 : xbsIndex_r4/Slice  nbits=3  boolean_output=off  mode=Lower Bit Location + Width  bit1=0  base1=MSB of Input  bit0=10  base0=LSB of Input  dbl_ovrd=off  block_type=slice
  Subsystem1 : Subsystem
  delay_bram_prog_dp : Subsystem  AncestorBlock=casper_library_delays/delay_bram_prog_dp  mask(delay_bram_prog_dp){ram_bits=max_delay_bits-3, bram_latency=2, async=off}
      mask prompts: ram_bits "Max delay (2^?)"; bram_latency "BRAM latency"; async "asynchronous operation"
      mask init:
      | delay_bram_prog_dp_init(gcb, ...
      |     'ram_bits', ram_bits, ...
      |     'bram_latency', bram_latency, ...
      |     'async', async);
  dout : Outport
  wires:
  Subsystem1/1(dout) -> dout/1
  delay_bram_prog_dp/1(dout) -> Subsystem1/1(din)
  Slice1/1 -> Subsystem1/2(delay)
  Slice/1 -> delay_bram_prog_dp/2(delay)
  delay/1 -> Slice/1, Slice1/1
  din/1 -> delay_bram_prog_dp/1(din)

== system delay_test/delay/Subsystem/3 ==
  din : Inport
  delay : Inport  Port=2
  Slice : xbsIndex_r4/Slice  nbits=10  boolean_output=off  mode=Lower Bit Location + Width  bit1=0  base1=MSB of Input  bit0=0  base0=LSB of Input  dbl_ovrd=off  block_type=slice
  Slice1 : xbsIndex_r4/Slice  nbits=3  boolean_output=off  mode=Lower Bit Location + Width  bit1=0  base1=MSB of Input  bit0=10  base0=LSB of Input  dbl_ovrd=off  block_type=slice
  Subsystem1 : Subsystem
  delay_bram_prog_dp : Subsystem  AncestorBlock=casper_library_delays/delay_bram_prog_dp  mask(delay_bram_prog_dp){ram_bits=max_delay_bits-3, bram_latency=2, async=off}
      mask prompts: ram_bits "Max delay (2^?)"; bram_latency "BRAM latency"; async "asynchronous operation"
      mask init:
      | delay_bram_prog_dp_init(gcb, ...
      |     'ram_bits', ram_bits, ...
      |     'bram_latency', bram_latency, ...
      |     'async', async);
  dout : Outport
  wires:
  Subsystem1/1(dout) -> dout/1
  delay_bram_prog_dp/1(dout) -> Subsystem1/1(din)
  Slice1/1 -> Subsystem1/2(delay)
  Slice/1 -> delay_bram_prog_dp/2(delay)
  delay/1 -> Slice/1, Slice1/1
  din/1 -> delay_bram_prog_dp/1(din)

== system delay_test/delay/Subsystem/30 ==
  din : Inport
  delay : Inport  Port=2
  Slice : xbsIndex_r4/Slice  nbits=10  boolean_output=off  mode=Lower Bit Location + Width  bit1=0  base1=MSB of Input  bit0=0  base0=LSB of Input  dbl_ovrd=off  block_type=slice
  Slice1 : xbsIndex_r4/Slice  nbits=3  boolean_output=off  mode=Lower Bit Location + Width  bit1=0  base1=MSB of Input  bit0=10  base0=LSB of Input  dbl_ovrd=off  block_type=slice
  Subsystem1 : Subsystem
  delay_bram_prog_dp : Subsystem  AncestorBlock=casper_library_delays/delay_bram_prog_dp  mask(delay_bram_prog_dp){ram_bits=max_delay_bits-3, bram_latency=2, async=off}
      mask prompts: ram_bits "Max delay (2^?)"; bram_latency "BRAM latency"; async "asynchronous operation"
      mask init:
      | delay_bram_prog_dp_init(gcb, ...
      |     'ram_bits', ram_bits, ...
      |     'bram_latency', bram_latency, ...
      |     'async', async);
  dout : Outport
  wires:
  din/1 -> delay_bram_prog_dp/1(din)
  delay/1 -> Slice1/1, Slice/1
  Slice/1 -> delay_bram_prog_dp/2(delay)
  Slice1/1 -> Subsystem1/2(delay)
  delay_bram_prog_dp/1(dout) -> Subsystem1/1(din)
  Subsystem1/1(dout) -> dout/1

== system delay_test/delay/Subsystem/31 ==
  din : Inport
  delay : Inport  Port=2
  Slice : xbsIndex_r4/Slice  nbits=10  boolean_output=off  mode=Lower Bit Location + Width  bit1=0  base1=MSB of Input  bit0=0  base0=LSB of Input  dbl_ovrd=off  block_type=slice
  Slice1 : xbsIndex_r4/Slice  nbits=3  boolean_output=off  mode=Lower Bit Location + Width  bit1=0  base1=MSB of Input  bit0=10  base0=LSB of Input  dbl_ovrd=off  block_type=slice
  Subsystem1 : Subsystem
  delay_bram_prog_dp : Subsystem  AncestorBlock=casper_library_delays/delay_bram_prog_dp  mask(delay_bram_prog_dp){ram_bits=max_delay_bits-3, bram_latency=2, async=off}
      mask prompts: ram_bits "Max delay (2^?)"; bram_latency "BRAM latency"; async "asynchronous operation"
      mask init:
      | delay_bram_prog_dp_init(gcb, ...
      |     'ram_bits', ram_bits, ...
      |     'bram_latency', bram_latency, ...
      |     'async', async);
  dout : Outport
  wires:
  Subsystem1/1(dout) -> dout/1
  delay_bram_prog_dp/1(dout) -> Subsystem1/1(din)
  Slice1/1 -> Subsystem1/2(delay)
  Slice/1 -> delay_bram_prog_dp/2(delay)
  delay/1 -> Slice/1, Slice1/1
  din/1 -> delay_bram_prog_dp/1(din)

== system delay_test/delay/Subsystem/32 ==
  din : Inport
  delay : Inport  Port=2
  Slice : xbsIndex_r4/Slice  nbits=10  boolean_output=off  mode=Lower Bit Location + Width  bit1=0  base1=MSB of Input  bit0=0  base0=LSB of Input  dbl_ovrd=off  block_type=slice
  Slice1 : xbsIndex_r4/Slice  nbits=3  boolean_output=off  mode=Lower Bit Location + Width  bit1=0  base1=MSB of Input  bit0=10  base0=LSB of Input  dbl_ovrd=off  block_type=slice
  Subsystem1 : Subsystem
  delay_bram_prog_dp : Subsystem  AncestorBlock=casper_library_delays/delay_bram_prog_dp  mask(delay_bram_prog_dp){ram_bits=max_delay_bits-3, bram_latency=2, async=off}
      mask prompts: ram_bits "Max delay (2^?)"; bram_latency "BRAM latency"; async "asynchronous operation"
      mask init:
      | delay_bram_prog_dp_init(gcb, ...
      |     'ram_bits', ram_bits, ...
      |     'bram_latency', bram_latency, ...
      |     'async', async);
  dout : Outport
  wires:
  din/1 -> delay_bram_prog_dp/1(din)
  delay/1 -> Slice1/1, Slice/1
  Slice/1 -> delay_bram_prog_dp/2(delay)
  Slice1/1 -> Subsystem1/2(delay)
  delay_bram_prog_dp/1(dout) -> Subsystem1/1(din)
  Subsystem1/1(dout) -> dout/1

== system delay_test/delay/Subsystem/33 ==
  din : Inport
  delay : Inport  Port=2
  Slice : xbsIndex_r4/Slice  nbits=10  boolean_output=off  mode=Lower Bit Location + Width  bit1=0  base1=MSB of Input  bit0=0  base0=LSB of Input  dbl_ovrd=off  block_type=slice
  Slice1 : xbsIndex_r4/Slice  nbits=3  boolean_output=off  mode=Lower Bit Location + Width  bit1=0  base1=MSB of Input  bit0=10  base0=LSB of Input  dbl_ovrd=off  block_type=slice
  Subsystem1 : Subsystem
  delay_bram_prog_dp : Subsystem  AncestorBlock=casper_library_delays/delay_bram_prog_dp  mask(delay_bram_prog_dp){ram_bits=max_delay_bits-3, bram_latency=2, async=off}
      mask prompts: ram_bits "Max delay (2^?)"; bram_latency "BRAM latency"; async "asynchronous operation"
      mask init:
      | delay_bram_prog_dp_init(gcb, ...
      |     'ram_bits', ram_bits, ...
      |     'bram_latency', bram_latency, ...
      |     'async', async);
  dout : Outport
  wires:
  Subsystem1/1(dout) -> dout/1
  delay_bram_prog_dp/1(dout) -> Subsystem1/1(din)
  Slice1/1 -> Subsystem1/2(delay)
  Slice/1 -> delay_bram_prog_dp/2(delay)
  delay/1 -> Slice/1, Slice1/1
  din/1 -> delay_bram_prog_dp/1(din)

== system delay_test/delay/Subsystem/34 ==
  din : Inport
  delay : Inport  Port=2
  Slice : xbsIndex_r4/Slice  nbits=10  boolean_output=off  mode=Lower Bit Location + Width  bit1=0  base1=MSB of Input  bit0=0  base0=LSB of Input  dbl_ovrd=off  block_type=slice
  Slice1 : xbsIndex_r4/Slice  nbits=3  boolean_output=off  mode=Lower Bit Location + Width  bit1=0  base1=MSB of Input  bit0=10  base0=LSB of Input  dbl_ovrd=off  block_type=slice
  Subsystem1 : Subsystem
  delay_bram_prog_dp : Subsystem  AncestorBlock=casper_library_delays/delay_bram_prog_dp  mask(delay_bram_prog_dp){ram_bits=max_delay_bits-3, bram_latency=2, async=off}
      mask prompts: ram_bits "Max delay (2^?)"; bram_latency "BRAM latency"; async "asynchronous operation"
      mask init:
      | delay_bram_prog_dp_init(gcb, ...
      |     'ram_bits', ram_bits, ...
      |     'bram_latency', bram_latency, ...
      |     'async', async);
  dout : Outport
  wires:
  din/1 -> delay_bram_prog_dp/1(din)
  delay/1 -> Slice1/1, Slice/1
  Slice/1 -> delay_bram_prog_dp/2(delay)
  Slice1/1 -> Subsystem1/2(delay)
  delay_bram_prog_dp/1(dout) -> Subsystem1/1(din)
  Subsystem1/1(dout) -> dout/1

== system delay_test/delay/Subsystem/35 ==
  din : Inport
  delay : Inport  Port=2
  Slice : xbsIndex_r4/Slice  nbits=10  boolean_output=off  mode=Lower Bit Location + Width  bit1=0  base1=MSB of Input  bit0=0  base0=LSB of Input  dbl_ovrd=off  block_type=slice
  Slice1 : xbsIndex_r4/Slice  nbits=3  boolean_output=off  mode=Lower Bit Location + Width  bit1=0  base1=MSB of Input  bit0=10  base0=LSB of Input  dbl_ovrd=off  block_type=slice
  Subsystem1 : Subsystem
  delay_bram_prog_dp : Subsystem  AncestorBlock=casper_library_delays/delay_bram_prog_dp  mask(delay_bram_prog_dp){ram_bits=max_delay_bits-3, bram_latency=2, async=off}
      mask prompts: ram_bits "Max delay (2^?)"; bram_latency "BRAM latency"; async "asynchronous operation"
      mask init:
      | delay_bram_prog_dp_init(gcb, ...
      |     'ram_bits', ram_bits, ...
      |     'bram_latency', bram_latency, ...
      |     'async', async);
  dout : Outport
  wires:
  Subsystem1/1(dout) -> dout/1
  delay_bram_prog_dp/1(dout) -> Subsystem1/1(din)
  Slice1/1 -> Subsystem1/2(delay)
  Slice/1 -> delay_bram_prog_dp/2(delay)
  delay/1 -> Slice/1, Slice1/1
  din/1 -> delay_bram_prog_dp/1(din)

== system delay_test/delay/Subsystem/36 ==
  din : Inport
  delay : Inport  Port=2
  Slice : xbsIndex_r4/Slice  nbits=10  boolean_output=off  mode=Lower Bit Location + Width  bit1=0  base1=MSB of Input  bit0=0  base0=LSB of Input  dbl_ovrd=off  block_type=slice
  Slice1 : xbsIndex_r4/Slice  nbits=3  boolean_output=off  mode=Lower Bit Location + Width  bit1=0  base1=MSB of Input  bit0=10  base0=LSB of Input  dbl_ovrd=off  block_type=slice
  Subsystem1 : Subsystem
  delay_bram_prog_dp : Subsystem  AncestorBlock=casper_library_delays/delay_bram_prog_dp  mask(delay_bram_prog_dp){ram_bits=max_delay_bits-3, bram_latency=2, async=off}
      mask prompts: ram_bits "Max delay (2^?)"; bram_latency "BRAM latency"; async "asynchronous operation"
      mask init:
      | delay_bram_prog_dp_init(gcb, ...
      |     'ram_bits', ram_bits, ...
      |     'bram_latency', bram_latency, ...
      |     'async', async);
  dout : Outport
  wires:
  din/1 -> delay_bram_prog_dp/1(din)
  delay/1 -> Slice1/1, Slice/1
  Slice/1 -> delay_bram_prog_dp/2(delay)
  Slice1/1 -> Subsystem1/2(delay)
  delay_bram_prog_dp/1(dout) -> Subsystem1/1(din)
  Subsystem1/1(dout) -> dout/1

== system delay_test/delay/Subsystem/37 ==
  din : Inport
  delay : Inport  Port=2
  Slice : xbsIndex_r4/Slice  nbits=10  boolean_output=off  mode=Lower Bit Location + Width  bit1=0  base1=MSB of Input  bit0=0  base0=LSB of Input  dbl_ovrd=off  block_type=slice
  Slice1 : xbsIndex_r4/Slice  nbits=3  boolean_output=off  mode=Lower Bit Location + Width  bit1=0  base1=MSB of Input  bit0=10  base0=LSB of Input  dbl_ovrd=off  block_type=slice
  Subsystem1 : Subsystem
  delay_bram_prog_dp : Subsystem  AncestorBlock=casper_library_delays/delay_bram_prog_dp  mask(delay_bram_prog_dp){ram_bits=max_delay_bits-3, bram_latency=2, async=off}
      mask prompts: ram_bits "Max delay (2^?)"; bram_latency "BRAM latency"; async "asynchronous operation"
      mask init:
      | delay_bram_prog_dp_init(gcb, ...
      |     'ram_bits', ram_bits, ...
      |     'bram_latency', bram_latency, ...
      |     'async', async);
  dout : Outport
  wires:
  Subsystem1/1(dout) -> dout/1
  delay_bram_prog_dp/1(dout) -> Subsystem1/1(din)
  Slice1/1 -> Subsystem1/2(delay)
  Slice/1 -> delay_bram_prog_dp/2(delay)
  delay/1 -> Slice/1, Slice1/1
  din/1 -> delay_bram_prog_dp/1(din)

== system delay_test/delay/Subsystem/38 ==
  din : Inport
  delay : Inport  Port=2
  Slice : xbsIndex_r4/Slice  nbits=10  boolean_output=off  mode=Lower Bit Location + Width  bit1=0  base1=MSB of Input  bit0=0  base0=LSB of Input  dbl_ovrd=off  block_type=slice
  Slice1 : xbsIndex_r4/Slice  nbits=3  boolean_output=off  mode=Lower Bit Location + Width  bit1=0  base1=MSB of Input  bit0=10  base0=LSB of Input  dbl_ovrd=off  block_type=slice
  Subsystem1 : Subsystem
  delay_bram_prog_dp : Subsystem  AncestorBlock=casper_library_delays/delay_bram_prog_dp  mask(delay_bram_prog_dp){ram_bits=max_delay_bits-3, bram_latency=2, async=off}
      mask prompts: ram_bits "Max delay (2^?)"; bram_latency "BRAM latency"; async "asynchronous operation"
      mask init:
      | delay_bram_prog_dp_init(gcb, ...
      |     'ram_bits', ram_bits, ...
      |     'bram_latency', bram_latency, ...
      |     'async', async);
  dout : Outport
  wires:
  Subsystem1/1(dout) -> dout/1
  delay_bram_prog_dp/1(dout) -> Subsystem1/1(din)
  Slice1/1 -> Subsystem1/2(delay)
  Slice/1 -> delay_bram_prog_dp/2(delay)
  delay/1 -> Slice/1, Slice1/1
  din/1 -> delay_bram_prog_dp/1(din)

== system delay_test/delay/Subsystem/39 ==
  din : Inport
  delay : Inport  Port=2
  Slice : xbsIndex_r4/Slice  nbits=10  boolean_output=off  mode=Lower Bit Location + Width  bit1=0  base1=MSB of Input  bit0=0  base0=LSB of Input  dbl_ovrd=off  block_type=slice
  Slice1 : xbsIndex_r4/Slice  nbits=3  boolean_output=off  mode=Lower Bit Location + Width  bit1=0  base1=MSB of Input  bit0=10  base0=LSB of Input  dbl_ovrd=off  block_type=slice
  Subsystem1 : Subsystem
  delay_bram_prog_dp : Subsystem  AncestorBlock=casper_library_delays/delay_bram_prog_dp  mask(delay_bram_prog_dp){ram_bits=max_delay_bits-3, bram_latency=2, async=off}
      mask prompts: ram_bits "Max delay (2^?)"; bram_latency "BRAM latency"; async "asynchronous operation"
      mask init:
      | delay_bram_prog_dp_init(gcb, ...
      |     'ram_bits', ram_bits, ...
      |     'bram_latency', bram_latency, ...
      |     'async', async);
  dout : Outport
  wires:
  din/1 -> delay_bram_prog_dp/1(din)
  delay/1 -> Slice1/1, Slice/1
  Slice/1 -> delay_bram_prog_dp/2(delay)
  Slice1/1 -> Subsystem1/2(delay)
  delay_bram_prog_dp/1(dout) -> Subsystem1/1(din)
  Subsystem1/1(dout) -> dout/1

== system delay_test/delay/Subsystem/4 ==
  din : Inport
  delay : Inport  Port=2
  Slice : xbsIndex_r4/Slice  nbits=10  boolean_output=off  mode=Lower Bit Location + Width  bit1=0  base1=MSB of Input  bit0=0  base0=LSB of Input  dbl_ovrd=off  block_type=slice
  Slice1 : xbsIndex_r4/Slice  nbits=3  boolean_output=off  mode=Lower Bit Location + Width  bit1=0  base1=MSB of Input  bit0=10  base0=LSB of Input  dbl_ovrd=off  block_type=slice
  Subsystem1 : Subsystem
  delay_bram_prog_dp : Subsystem  AncestorBlock=casper_library_delays/delay_bram_prog_dp  mask(delay_bram_prog_dp){ram_bits=max_delay_bits-3, bram_latency=2, async=off}
      mask prompts: ram_bits "Max delay (2^?)"; bram_latency "BRAM latency"; async "asynchronous operation"
      mask init:
      | delay_bram_prog_dp_init(gcb, ...
      |     'ram_bits', ram_bits, ...
      |     'bram_latency', bram_latency, ...
      |     'async', async);
  dout : Outport
  wires:
  din/1 -> delay_bram_prog_dp/1(din)
  delay/1 -> Slice1/1, Slice/1
  Slice/1 -> delay_bram_prog_dp/2(delay)
  Slice1/1 -> Subsystem1/2(delay)
  delay_bram_prog_dp/1(dout) -> Subsystem1/1(din)
  Subsystem1/1(dout) -> dout/1

== system delay_test/delay/Subsystem/40 ==
  din : Inport
  delay : Inport  Port=2
  Slice : xbsIndex_r4/Slice  nbits=10  boolean_output=off  mode=Lower Bit Location + Width  bit1=0  base1=MSB of Input  bit0=0  base0=LSB of Input  dbl_ovrd=off  block_type=slice
  Slice1 : xbsIndex_r4/Slice  nbits=3  boolean_output=off  mode=Lower Bit Location + Width  bit1=0  base1=MSB of Input  bit0=10  base0=LSB of Input  dbl_ovrd=off  block_type=slice
  Subsystem1 : Subsystem
  delay_bram_prog_dp : Subsystem  AncestorBlock=casper_library_delays/delay_bram_prog_dp  mask(delay_bram_prog_dp){ram_bits=max_delay_bits-3, bram_latency=2, async=off}
      mask prompts: ram_bits "Max delay (2^?)"; bram_latency "BRAM latency"; async "asynchronous operation"
      mask init:
      | delay_bram_prog_dp_init(gcb, ...
      |     'ram_bits', ram_bits, ...
      |     'bram_latency', bram_latency, ...
      |     'async', async);
  dout : Outport
  wires:
  Subsystem1/1(dout) -> dout/1
  delay_bram_prog_dp/1(dout) -> Subsystem1/1(din)
  Slice1/1 -> Subsystem1/2(delay)
  Slice/1 -> delay_bram_prog_dp/2(delay)
  delay/1 -> Slice/1, Slice1/1
  din/1 -> delay_bram_prog_dp/1(din)
